simulink model "foc_current_estimator_test"  (R2021b)
settings: Solver=FixedStepDiscrete  StartTime=0.0  StopTime=6  FixedStep=Tsw  RelTol=1e-3
undefined symbols (not defined in the file): B, current_ki, current_kp, DiscIntNeverNeededParam, Ibase, id_ref, iq_ref, J, k1_sta, k2_sta, Ks, load_torque, Ls, qpll, Rs, sigmoid_a, speed_ki, speed_kp, Ts_speed, Tsw, Vbase, Vdc, w_base
libraries: mcbcontrolslib x6, simulink_extras x2, mcbplantlib x1, autolibpmsmexterior x1
settings Model: Creator=gary  LastModifiedBy=goldf
settings DebuggingCC: SFMachineParentedDataDiag=warning

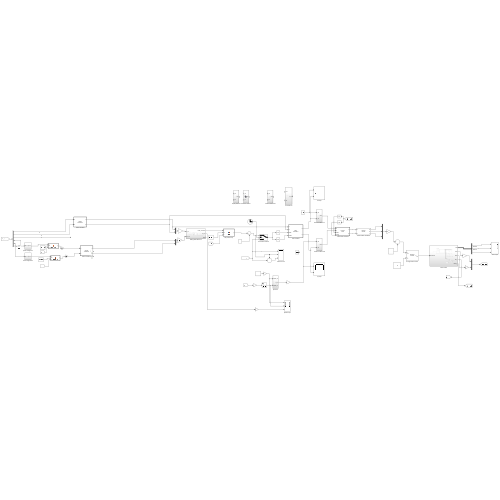
[thumbnail: Simulink's stored preview of the top-level diagram]
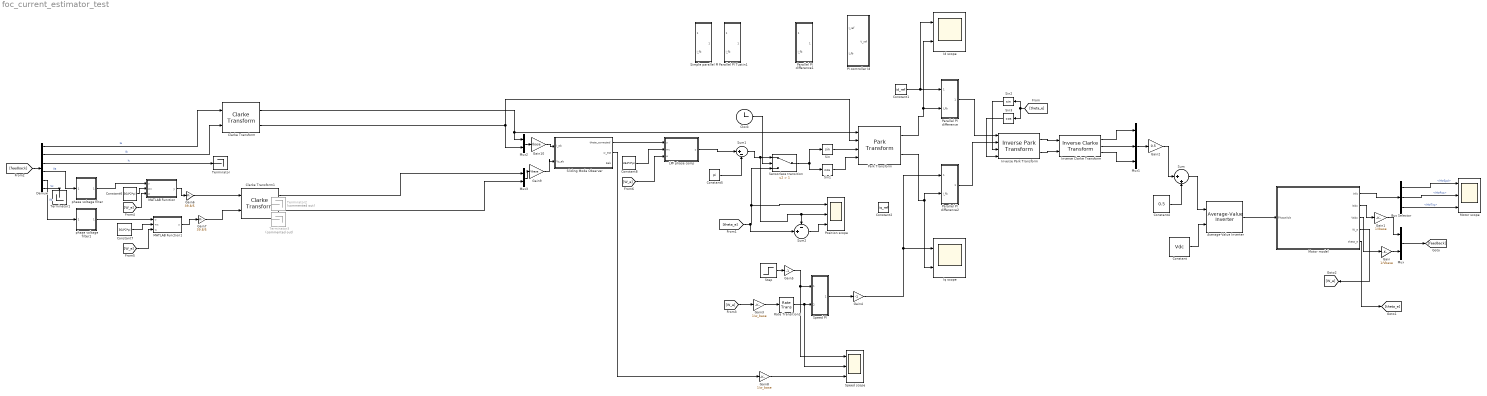
== system foc_current_estimator_test ==
  Average-Value Inverter : mcbplantlib/Average-Value Inverter
  Bus Selector : BusSelector  OutputSignals=MtrSpd,MtrPos,MtrTrq
  Clarke Transform : mcbcontrolslib/Clarke Transform  VariantControl=Variant2
  Clarke Transform1 : mcbcontrolslib/Clarke Transform  VariantControl=Variant2
  Clock : Clock
  Constant : Constant  Value=Vdc
  Constant1 : Constant  Value=id_ref
  Constant2 : Constant  Value=iq_ref
  Constant4 : Constant  Value=0.5
  Constant5 : Constant  Value=pi
  Constant6 : Constant  Value=364*2*pi
  Constant7 : Constant  Value=364*2*pi
  Constant8 : Constant  Value=364*2*pi
  Demux : Demux  Outputs=6
  Gain : Gain  Gain=1/Vbase
  Gain1 : Gain  Gain=1/Ibase
  Gain10 : Gain  Gain=Ibase
  Gain2 : Gain  Gain=0.5
  Gain3 : Gain  Gain=1/w_base
  Gain4 : Gain  Gain=-1
  Gain5 : Gain  Gain=-1
  Gain6 : Gain  Gain=39.8/5
  Gain7 : Gain  Gain=39.8/5
  Gain8 : Gain  Gain=1/w_base
  Gain9 : Gain  Gain=Vbase
  Id scope : Scope  NumInputPorts=2
  Inverse Clarke Transform : mcbcontrolslib/Inverse Clarke Transform
      settings: SourceProductBaseCode=MT
  Inverse Park Transform : mcbcontrolslib/Inverse Park Transform  AxisAlignment=D-axis
  Iq scope : Scope  NumInputPorts=2
  LPF phase comp : MATLAB Function  TreatAsAtomicUnit=on
  MATLAB Function : MATLAB Function  TreatAsAtomicUnit=on
  MATLAB Function1 : MATLAB Function  TreatAsAtomicUnit=on
  Motor model : Subsystem
  Motor scope : Scope  NumInputPorts=3
  Mux : Mux  Inputs=2
  Mux1 : Mux  Inputs=3
  Mux2 : Mux  Inputs=2
  Mux3 : Mux  Inputs=2
  PI controller Id : Subsystem
  Parallel PI Tustin1 : Subsystem
  Parallel PI difference : Subsystem
  Parallel PI difference1 : Subsystem
  Parallel PI difference2 : Subsystem
  Park Transform : mcbcontrolslib/Park Transform  AxisAlignment=D-axis
      settings: SourceProductBaseCode=MT
  Position scope : Scope  NumInputPorts=3
  Rate Transition2 : RateTransition  OutPortSampleTime=Ts_speed
  Sensorless transition : Switch  Criteria=u2 > Threshold  Threshold=1
  Simple parallel PI : Subsystem
  Sin : Trigonometry
  Sin1 : Trigonometry  Operator=cos
  Sin2 : Trigonometry
  Sin3 : Trigonometry  Operator=cos
  Sliding Mode Observer : Subsystem
  Speed PI : Subsystem
  Speed scope : Scope  NumInputPorts=3
  Step : Step  Time=3  Before=0.4  After=0.4  SampleTime=0
  Sum : Sum  Inputs=|++
  Sum1 : Sum  Inputs=|+-
  Sum2 : Sum  Inputs=-+|
  Terminator : Terminator
  Terminator1 : Terminator
  Terminator2 : Terminator  Commented=on
  Terminator3 : Terminator  Commented=on
  phase voltage filter : Subsystem
  phase voltage filter1 : Subsystem
  wires:
  Constant/1 -> Average-Value Inverter/2
  Motor model/1(Info) -> Bus Selector/1
  Bus Selector/2 -> Motor scope/2  "<MtrPos>"
  Bus Selector/3 -> Motor scope/3  "<MtrTrq>"
  Mux/1 -> [feedback]
  [feedback] -> Demux/1
  Demux/3 -> Terminator/1  "Ic"
  Demux/1 -> Clarke Transform/1  "Ia"
  Demux/2 -> Clarke Transform/2  "Ib"
  Park Transform/1 -> Parallel PI difference/2(I_fb), Id scope/2
  Park Transform/2 -> Parallel PI difference2/2(I_fb), Iq scope/2
  Constant1/1 -> Parallel PI difference/1(I_ref), Id scope/1
  Parallel PI difference/1(Vref) -> Inverse Park Transform/1
  Parallel PI difference2/1(Vref) -> Inverse Park Transform/2
  [theta_e] -> Sin2/1, Sin3/1
  Sin2/1 -> Inverse Park Transform/3
  Sin3/1 -> Inverse Park Transform/4
  Inverse Park Transform/1 -> Inverse Clarke Transform/1
  Inverse Park Transform/2 -> Inverse Clarke Transform/2
  Inverse Clarke Transform/2 -> Mux1/2
  Inverse Clarke Transform/3 -> Mux1/3
  Inverse Clarke Transform/1 -> Mux1/1
  Average-Value Inverter/1 -> Motor model/1(PhaseVolt)
  Motor model/2(Iabc) -> Gain1/1
  Gain1/1 -> Mux/1
  Motor model/3(Vabc) -> Gain/1
  Demux/6 -> Terminator1/1  "Vc"
  Clarke Transform/1 -> Mux2/1, Park Transform/1
  Clarke Transform/2 -> Mux2/2, Park Transform/2
  Sin/1 -> Park Transform/3
  Sin1/1 -> Park Transform/4
  Motor model/5(theta_e) -> [theta_e]
  Gain/1 -> Mux/2
  Mux1/1 -> Gain2/1
  Gain2/1 -> Sum/1
  Sum/1 -> Average-Value Inverter/1
  Constant4/1 -> Sum/2
  [theta_e] -> Sum2/2, Position scope/1, Sensorless transition/3
  Bus Selector/1 -> Motor scope/1  "<MtrSpd>"
  Clock/1 -> Sensorless transition/2
  Sensorless transition/1 -> Sin1/1, Sin/1
  Sum1/1 -> Sum2/1, Position scope/2, Sensorless transition/1
  Constant5/1 -> Sum1/2
  [W_e] -> Gain3/1
  Gain5/1 -> Speed scope/1, Speed PI/1(Speed_ref)
  Rate Transition2/1 -> Speed scope/2, Speed PI/2(Speed_fb)
  Step/1 -> Gain5/1
  Speed PI/1(I_ref) -> Gain4/1
  Gain3/1 -> Rate Transition2/1
  Motor model/4(W_e) -> [W_e]
  Gain4/1 -> Parallel PI difference2/1(I_ref), Iq scope/1
  [W_e] -> MATLAB Function/3(w)
  Constant6/1 -> MATLAB Function/2(wc)
  MATLAB Function/1(y) -> Gain6/1
  phase voltage filter/1(lpf out) -> MATLAB Function/1(u)
  phase voltage filter1/1(lpf out) -> MATLAB Function1/1(u)
  Constant7/1 -> MATLAB Function1/2(wc)
  [W_e] -> MATLAB Function1/3(w)
  MATLAB Function1/1(y) -> Gain7/1
  Demux/4 -> phase voltage filter/1(lpf in)  "Va"
  Demux/5 -> phase voltage filter1/1(lpf in)  "Vb"
  Constant8/1 -> LPF phase comp/2(wc)
  [W_e] -> LPF phase comp/3(w)
  Sliding Mode Observer/2(w_est) -> Gain8/1
  Gain8/1 -> Speed scope/3
  Mux2/1 -> Gain10/1
  Gain10/1 -> Sliding Mode Observer/1(I_ab)
  Mux3/1 -> Gain9/1
  Gain9/1 -> Sliding Mode Observer/2(Vs_ab)
  Sum2/1 -> Position scope/3
  Clarke Transform1/1 -> Mux3/1
  Clarke Transform1/2 -> Mux3/2
  Gain6/1 -> Clarke Transform1/1
  Gain7/1 -> Clarke Transform1/2
  Sliding Mode Observer/1(theta_corrected) -> LPF phase comp/1(u)
  LPF phase comp/1(y) -> Sum1/1

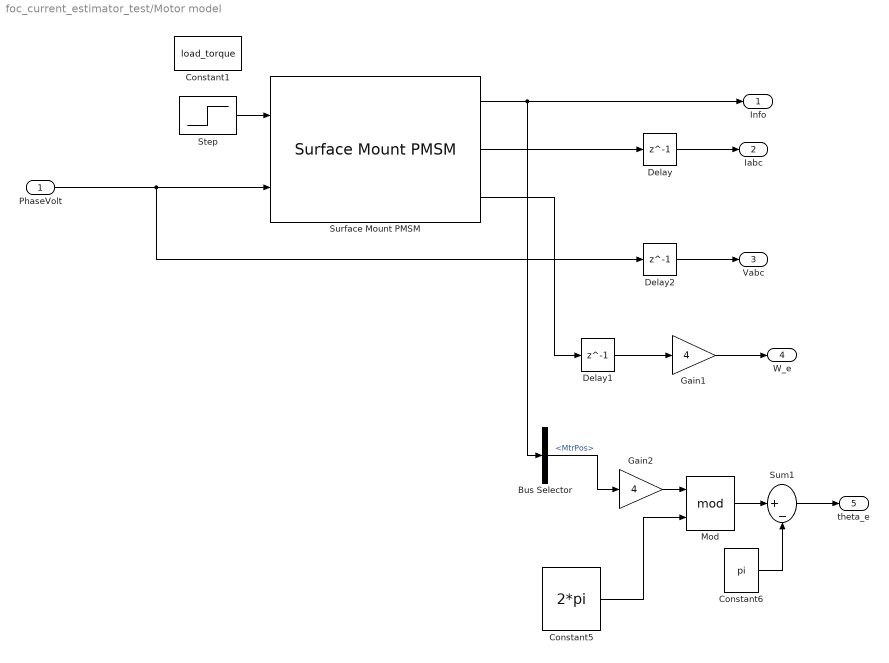
== system foc_current_estimator_test/Motor model ==
  PhaseVolt : Inport
  Bus Selector : BusSelector  OutputSignals=MtrPos
  Constant1 : Constant  Value=load_torque
  Constant5 : Constant  Value=2*pi
  Constant6 : Constant  Value=pi
  Delay : Delay  DelayLength=1  InitialCondition=0
  Delay1 : Delay  DelayLength=1  InitialCondition=0
  Delay2 : Delay  DelayLength=1  InitialCondition=0
  Gain1 : Gain  Gain=4
  Gain2 : Gain  Gain=4
  Mod : Math  Operator=mod  SaturateOnIntegerOverflow=on
  Step : Step  Time=3  Before=-0.02  After=-0.4  SampleTime=0
  Sum1 : Sum  Inputs=|+-
  Surface Mount PMSM : autolibpmsmexterior/Surface Mount PMSM  port_config=Torque  sim_type=Discrete  Ts=Tsw  P=4  Rs=1.5*Rs  Ldq_=0.3*Ls  KConstText=Permanent flux linkage constant (lambda_pm):  lambda_pm=lambda  Ke=159.9771  Kt=1.323  mechanical=[J, B, 0]  idq0=[0 0]  theta_init=0  omega_init=-100  KConst=lambda  lambda_pm_calc=lambda  RefBlkName='autolibpmsmexterior/Surface Mount PMSM'  aMode=5  Ldq="[0.0017      0.0017]"
      settings: SourceProductBaseCode=PW,DR,MT,UV,VE
  Info : Outport
  Iabc : Outport  Port=2
  Vabc : Outport  Port=3
  W_e : Outport  Port=4
  theta_e : Outport  Port=5
  wires:
  Surface Mount PMSM/1 -> Info/1, Bus Selector/1
  Surface Mount PMSM/2 -> Delay/1
  PhaseVolt/1 -> Delay2/1, Surface Mount PMSM/2
  Step/1 -> Surface Mount PMSM/1
  Surface Mount PMSM/3 -> Delay1/1
  Delay/1 -> Iabc/1
  Bus Selector/1 -> Gain2/1  "<MtrPos>"
  Gain2/1 -> Mod/1
  Constant5/1 -> Mod/2
  Sum1/1 -> theta_e/1
  Mod/1 -> Sum1/1
  Constant6/1 -> Sum1/2
  Delay1/1 -> Gain1/1
  Gain1/1 -> W_e/1
  Delay2/1 -> Vabc/1

== system foc_current_estimator_test/PI controller Id ==
  I_ref : Inport
  I_fb : Inport  Port=2
  Constant1 : Constant  Value=0
  Constant2 : Constant  Value=current_kp
  Constant3 : Constant  Value=current_ki*Tsw
  Constant4 : Constant  Value=0
  Discrete PI Controller with anti-windup & reset : mcbcontrolslib/Discrete PI Controller  with anti-windup & reset  UpperSaturationLimit=1  LowerSaturationLimit=-1
      settings: SourceProductBaseCode=MT
  Sum : Sum  Inputs=|+-
  V_ref : Outport
  wires:
  I_ref/1 -> Sum/1
  Constant4/1 -> Discrete PI Controller with anti-windup & reset/5
  Discrete PI Controller with anti-windup & reset/1 -> V_ref/1
  Constant1/1 -> Discrete PI Controller with anti-windup & reset/4
  I_fb/1 -> Sum/2
  Constant2/1 -> Discrete PI Controller with anti-windup & reset/2
  Sum/1 -> Discrete PI Controller with anti-windup & reset/1
  Constant3/1 -> Discrete PI Controller with anti-windup & reset/3

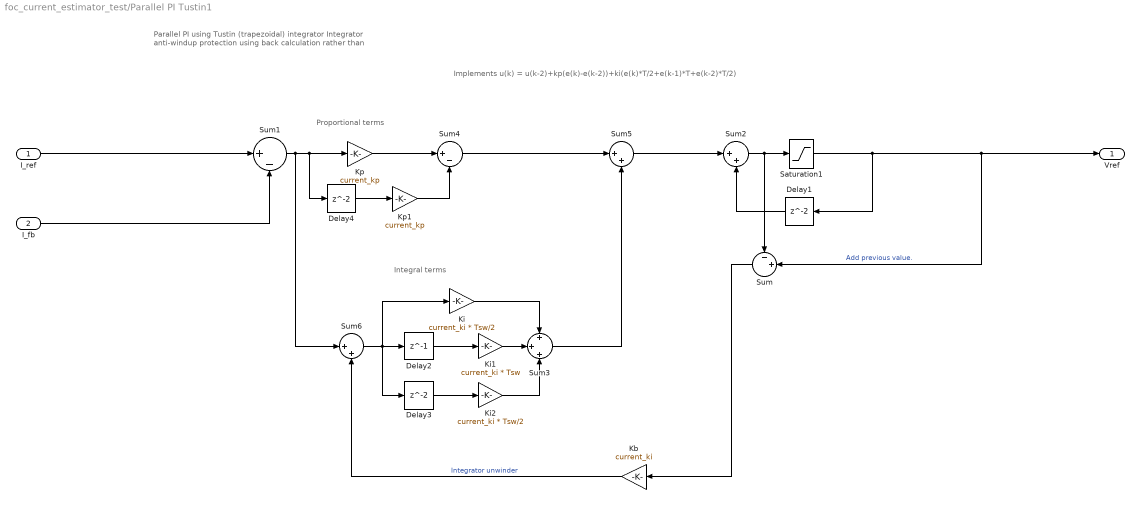
== system foc_current_estimator_test/Parallel PI Tustin1 ==
  note: Implements u(k) = u(k-2)+kp(e(k)-e(k-2))+ki(e(k)*T/2+e(k-1)*T+e(k-2)*T/2)
  note: Integral terms
  note: Proportional terms
  note: Parallel PI using Tustin (trapezoidal) integrator
      | Integrator anti-windup protection using back calculation
      | rather than
  I_ref : Inport
  I_fb : Inport  Port=2
  Delay1 : Delay  InitialCondition=0
  Delay2 : Delay  DelayLength=1  InitialCondition=0
  Delay3 : Delay  InitialCondition=0
  Delay4 : Delay  InitialCondition=0
  Kb : Gain  Gain=current_ki
  Ki : Gain  Gain=current_ki * Tsw/2
  Ki1 : Gain  Gain=current_ki * Tsw
  Ki2 : Gain  Gain=current_ki * Tsw/2
  Kp : Gain  Gain=current_kp
  Kp1 : Gain  Gain=current_kp
  Saturation1 : Saturate  UpperLimit=1  LowerLimit=-1
  Sum : Sum  Inputs=-+|
  Sum1 : Sum  Inputs=|+-
  Sum2 : Sum  Inputs=|++
  Sum3 : Sum  Inputs=+|+|+
  Sum4 : Sum  Inputs=|+-
  Sum5 : Sum  Inputs=|++
  Sum6 : Sum  Inputs=|++
  Vref : Outport
  wires:
  Sum1/1 -> Sum6/1, Delay4/1, Kp/1
  I_fb/1 -> Sum1/2
  I_ref/1 -> Sum1/1
  Kp/1 -> Sum4/1
  Delay1/1 -> Sum2/2
  Sum2/1 -> Sum/1, Saturation1/1
  Sum/1 -> Kb/1
  Delay2/1 -> Ki1/1
  Delay3/1 -> Ki2/1
  Delay4/1 -> Kp1/1
  Kp1/1 -> Sum4/2
  Ki1/1 -> Sum3/2
  Ki/1 -> Sum3/1
  Ki2/1 -> Sum3/3
  Sum4/1 -> Sum5/1
  Sum6/1 -> Delay3/1, Delay2/1, Ki/1
  Sum3/1 -> Sum5/2
  Sum5/1 -> Sum2/1
  Kb/1 -> Sum6/2  "Integrator unwinder"
  Saturation1/1 -> Sum/2, Vref/1, Delay1/1  "Add previous value."

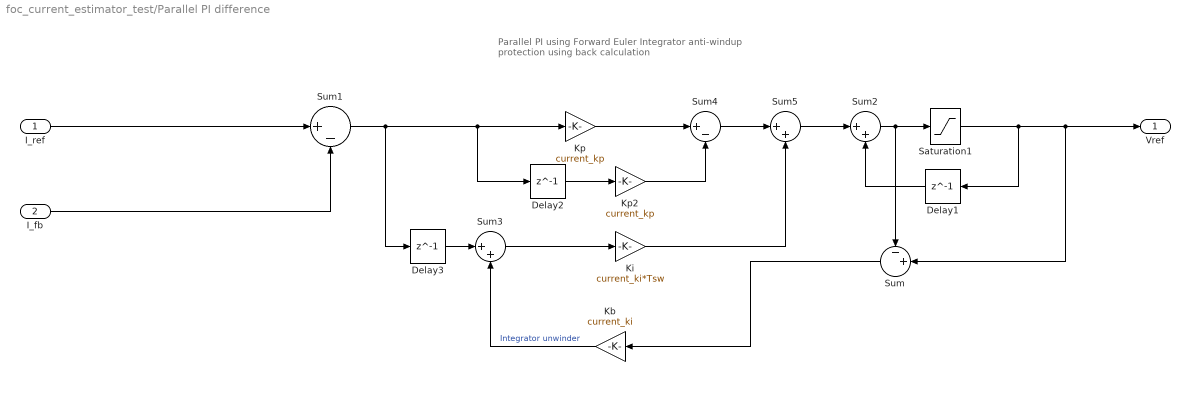
== system foc_current_estimator_test/Parallel PI difference ==
  note: Parallel PI using Forward Euler
      | Integrator anti-windup protection using back calculation
  I_ref : Inport
  I_fb : Inport  Port=2
  Delay1 : Delay  DelayLength=1  InitialCondition=0
  Delay2 : Delay  DelayLength=1  InitialCondition=0
  Delay3 : Delay  DelayLength=1  InitialCondition=0
  Kb : Gain  Gain=current_ki
  Ki : Gain  Gain=current_ki*Tsw
  Kp : Gain  Gain=current_kp
  Kp2 : Gain  Gain=current_kp
  Saturation1 : Saturate  UpperLimit=1  LowerLimit=0
  Sum : Sum  Inputs=-+|
  Sum1 : Sum  Inputs=|+-
  Sum2 : Sum  Inputs=|++
  Sum3 : Sum  Inputs=|++
  Sum4 : Sum  Inputs=|+-
  Sum5 : Sum  Inputs=|++
  Vref : Outport
  wires:
  I_fb/1 -> Sum1/2
  I_ref/1 -> Sum1/1
  Sum1/1 -> Delay2/1, Kp/1, Delay3/1
  Kp/1 -> Sum4/1
  Delay1/1 -> Sum2/2
  Sum2/1 -> Saturation1/1, Sum/1
  Saturation1/1 -> Sum/2, Vref/1, Delay1/1
  Kb/1 -> Sum3/2  "Integrator unwinder"
  Sum/1 -> Kb/1
  Delay2/1 -> Kp2/1
  Kp2/1 -> Sum4/2
  Sum3/1 -> Ki/1
  Delay3/1 -> Sum3/1
  Sum4/1 -> Sum5/1
  Ki/1 -> Sum5/2
  Sum5/1 -> Sum2/1

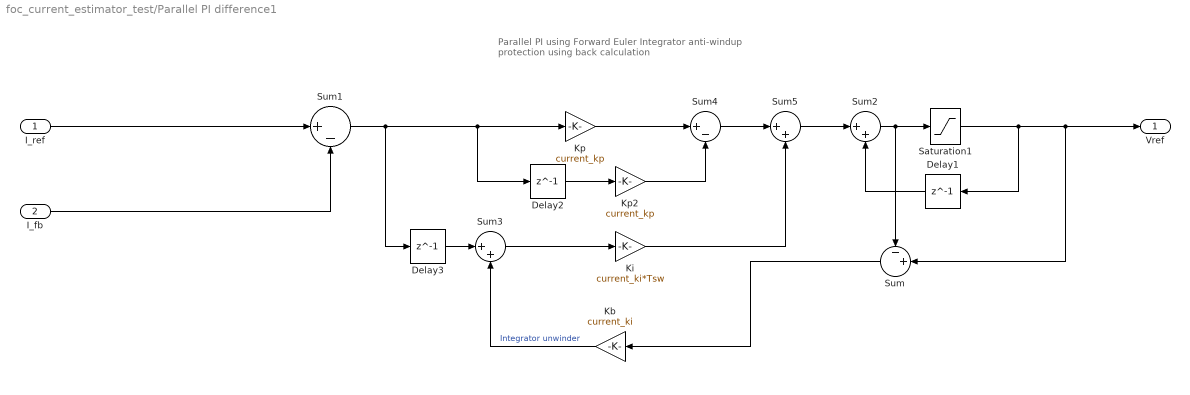
== system foc_current_estimator_test/Parallel PI difference1 ==
  note: Parallel PI using Forward Euler
      | Integrator anti-windup protection using back calculation
  I_ref : Inport
  I_fb : Inport  Port=2
  Delay1 : Delay  DelayLength=1  InitialCondition=0
  Delay2 : Delay  DelayLength=1  InitialCondition=0
  Delay3 : Delay  DelayLength=1  InitialCondition=0
  Kb : Gain  Gain=current_ki
  Ki : Gain  Gain=current_ki*Tsw
  Kp : Gain  Gain=current_kp
  Kp2 : Gain  Gain=current_kp
  Saturation1 : Saturate  UpperLimit=1  LowerLimit=0
  Sum : Sum  Inputs=-+|
  Sum1 : Sum  Inputs=|+-
  Sum2 : Sum  Inputs=|++
  Sum3 : Sum  Inputs=|++
  Sum4 : Sum  Inputs=|+-
  Sum5 : Sum  Inputs=|++
  Vref : Outport
  wires:
  I_fb/1 -> Sum1/2
  I_ref/1 -> Sum1/1
  Sum1/1 -> Delay2/1, Kp/1, Delay3/1
  Kp/1 -> Sum4/1
  Delay1/1 -> Sum2/2
  Sum2/1 -> Saturation1/1, Sum/1
  Saturation1/1 -> Sum/2, Vref/1, Delay1/1
  Kb/1 -> Sum3/2  "Integrator unwinder"
  Sum/1 -> Kb/1
  Delay2/1 -> Kp2/1
  Kp2/1 -> Sum4/2
  Sum3/1 -> Ki/1
  Delay3/1 -> Sum3/1
  Sum4/1 -> Sum5/1
  Ki/1 -> Sum5/2
  Sum5/1 -> Sum2/1

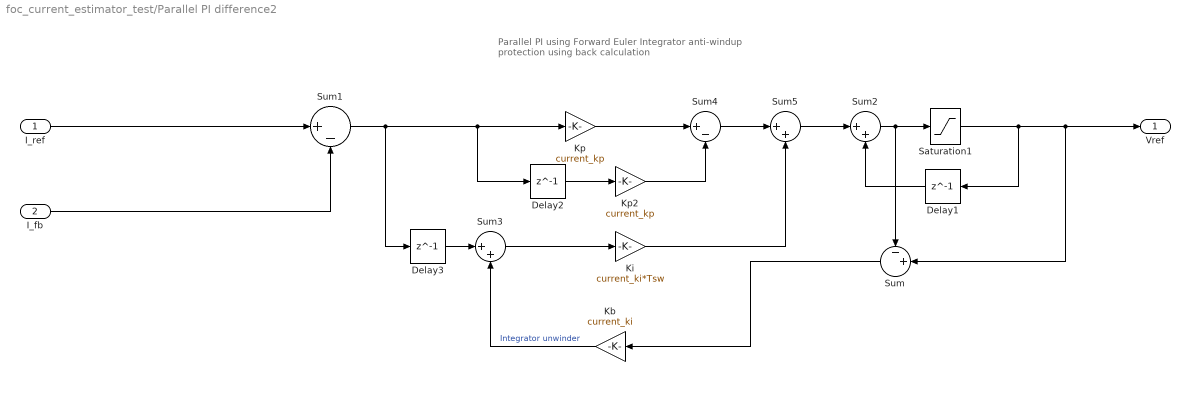
== system foc_current_estimator_test/Parallel PI difference2 ==
  note: Parallel PI using Forward Euler
      | Integrator anti-windup protection using back calculation
  I_ref : Inport
  I_fb : Inport  Port=2
  Delay1 : Delay  DelayLength=1  InitialCondition=0
  Delay2 : Delay  DelayLength=1  InitialCondition=0
  Delay3 : Delay  DelayLength=1  InitialCondition=0
  Kb : Gain  Gain=current_ki
  Ki : Gain  Gain=current_ki*Tsw
  Kp : Gain  Gain=current_kp
  Kp2 : Gain  Gain=current_kp
  Saturation1 : Saturate  UpperLimit=1  LowerLimit=0
  Sum : Sum  Inputs=-+|
  Sum1 : Sum  Inputs=|+-
  Sum2 : Sum  Inputs=|++
  Sum3 : Sum  Inputs=|++
  Sum4 : Sum  Inputs=|+-
  Sum5 : Sum  Inputs=|++
  Vref : Outport
  wires:
  I_fb/1 -> Sum1/2
  I_ref/1 -> Sum1/1
  Sum1/1 -> Delay2/1, Kp/1, Delay3/1
  Kp/1 -> Sum4/1
  Delay1/1 -> Sum2/2
  Sum2/1 -> Saturation1/1, Sum/1
  Saturation1/1 -> Sum/2, Vref/1, Delay1/1
  Kb/1 -> Sum3/2  "Integrator unwinder"
  Sum/1 -> Kb/1
  Delay2/1 -> Kp2/1
  Kp2/1 -> Sum4/2
  Sum3/1 -> Ki/1
  Delay3/1 -> Sum3/1
  Sum4/1 -> Sum5/1
  Ki/1 -> Sum5/2
  Sum5/1 -> Sum2/1

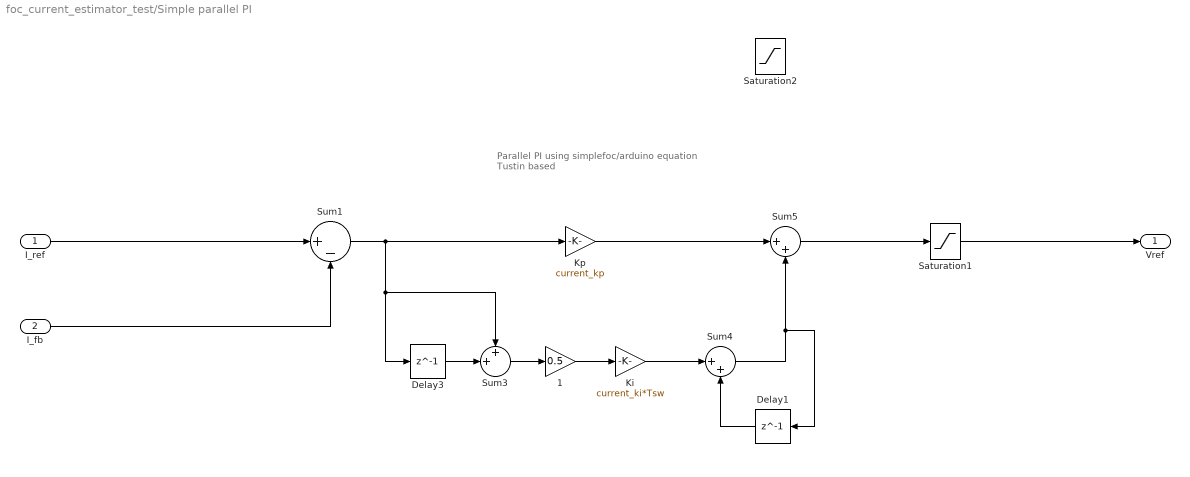
== system foc_current_estimator_test/Simple parallel PI ==
  note: Parallel PI using simplefoc/arduino equation
      | Tustin based
  I_ref : Inport
  I_fb : Inport  Port=2
  1 : Gain  Gain=0.5
  Delay1 : Delay  DelayLength=1  InitialCondition=0
  Delay3 : Delay  DelayLength=1  InitialCondition=0
  Ki : Gain  Gain=current_ki*Tsw
  Kp : Gain  Gain=current_kp
  Saturation1 : Saturate  UpperLimit=1  LowerLimit=0
  Saturation2 : Saturate  UpperLimit=1  LowerLimit=0
  Sum1 : Sum  Inputs=|+-
  Sum3 : Sum  Inputs=++|
  Sum4 : Sum  Inputs=|++
  Sum5 : Sum  Inputs=|++
  Vref : Outport
  wires:
  I_fb/1 -> Sum1/2
  I_ref/1 -> Sum1/1
  Sum5/1 -> Saturation1/1
  Saturation1/1 -> Vref/1
  Sum3/1 -> 1/1
  Kp/1 -> Sum5/1
  Delay3/1 -> Sum3/2
  Sum1/1 -> Kp/1, Sum3/1, Delay3/1
  1/1 -> Ki/1
  Ki/1 -> Sum4/1
  Sum4/1 -> Delay1/1, Sum5/2
  Delay1/1 -> Sum4/2

== system foc_current_estimator_test/Sliding Mode Observer ==
  I_ab : Inport
  Vs_ab : Inport  Port=2
  Constant10 : Constant  Value=qpll.kp
  Constant9 : Constant  Value=qpll.ki
  Demux1 : Demux  Outputs=2
  QPLL : Subsystem
  Reversal 180 phase shift : Subsystem
  SMO bemf estimator1 : Subsystem
  SMO bemf estimator3 : Subsystem  Commented=on
  theta_corrected : Outport
  w_est : Outport  Port=2
  Eab : Outport  Port=3
  wires:
  SMO bemf estimator1/1(E_ab) -> Eab/1, Demux1/1
  Reversal 180 phase shift/1(theta_corrected) -> theta_corrected/1
  Constant9/1 -> QPLL/2(ki)
  Vs_ab/1 -> SMO bemf estimator1/2(Vs_ab)
  QPLL/1(theta_est) -> Reversal 180 phase shift/1(theta_uncorrected)
  Constant10/1 -> QPLL/1(kp)
  QPLL/2(w) -> w_est/1, Reversal 180 phase shift/2(W_est)
  Demux1/2 -> QPLL/4(E_beta)
  Demux1/1 -> QPLL/3(E_alpha)
  I_ab/1 -> SMO bemf estimator1/1(I_ab)

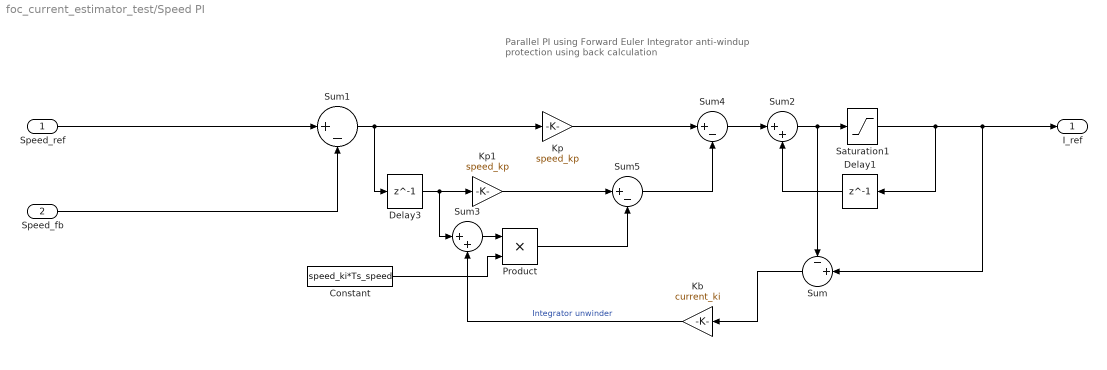
== system foc_current_estimator_test/Speed PI ==
  note: Parallel PI using Forward Euler
      | Integrator anti-windup protection using back calculation
  Speed_ref : Inport
  Speed_fb : Inport  Port=2
  Constant : Constant  Value=speed_ki*Ts_speed
  Delay1 : Delay  DelayLength=1  InitialCondition=0
  Delay3 : Delay  DelayLength=1  InitialCondition=0
  Kb : Gain  Gain=current_ki
  Kp : Gain  Gain=speed_kp
  Kp1 : Gain  Gain=speed_kp
  Product : Product
  Saturation1 : Saturate  UpperLimit=1  LowerLimit=-1
  Sum : Sum  Inputs=-+|
  Sum1 : Sum  Inputs=|+-
  Sum2 : Sum  Inputs=|++
  Sum3 : Sum  Inputs=|++
  Sum4 : Sum  Inputs=|+-
  Sum5 : Sum  Inputs=|+-
  I_ref : Outport
  wires:
  Sum1/1 -> Delay3/1, Kp/1
  Speed_fb/1 -> Sum1/2
  Speed_ref/1 -> Sum1/1
  Constant/1 -> Product/2
  Delay3/1 -> Kp1/1, Sum3/1
  Kp1/1 -> Sum5/1
  Kp/1 -> Sum4/1
  Delay1/1 -> Sum2/2
  Sum4/1 -> Sum2/1
  Sum2/1 -> Sum/1, Saturation1/1
  Sum5/1 -> Sum4/2
  Product/1 -> Sum5/2
  Sum3/1 -> Product/1
  Kb/1 -> Sum3/2  "Integrator unwinder"
  Sum/1 -> Kb/1
  Saturation1/1 -> Sum/2, I_ref/1, Delay1/1

== system foc_current_estimator_test/phase voltage filter ==
  lpf in : Inport
  Instaspin lpf tf : simulink_extras/Additional Discrete/Discrete Transfer Fcn (with initial outputs)  N=[0.006918, 0.006659]  D=[1 -0.8919]  U0=[1]  Y0=0  TS=-1
      settings: SourceProductBaseCode=SL
  Rate Transition1 : RateTransition  OutPortSampleTime=Tsw
  lpf out : Outport
  wires:
  Rate Transition1/1 -> Instaspin lpf tf/1
  Instaspin lpf tf/1 -> lpf out/1
  lpf in/1 -> Rate Transition1/1

== system foc_current_estimator_test/phase voltage filter1 ==
  lpf in : Inport
  Instaspin lpf tf : simulink_extras/Additional Discrete/Discrete Transfer Fcn (with initial outputs)  N=[0.006918, 0.006659]  D=[1 -0.8919]  U0=[1]  Y0=0  TS=-1
      settings: SourceProductBaseCode=SL
  Rate Transition1 : RateTransition  OutPortSampleTime=Tsw
  lpf out : Outport
  wires:
  Rate Transition1/1 -> Instaspin lpf tf/1
  Instaspin lpf tf/1 -> lpf out/1
  lpf in/1 -> Rate Transition1/1

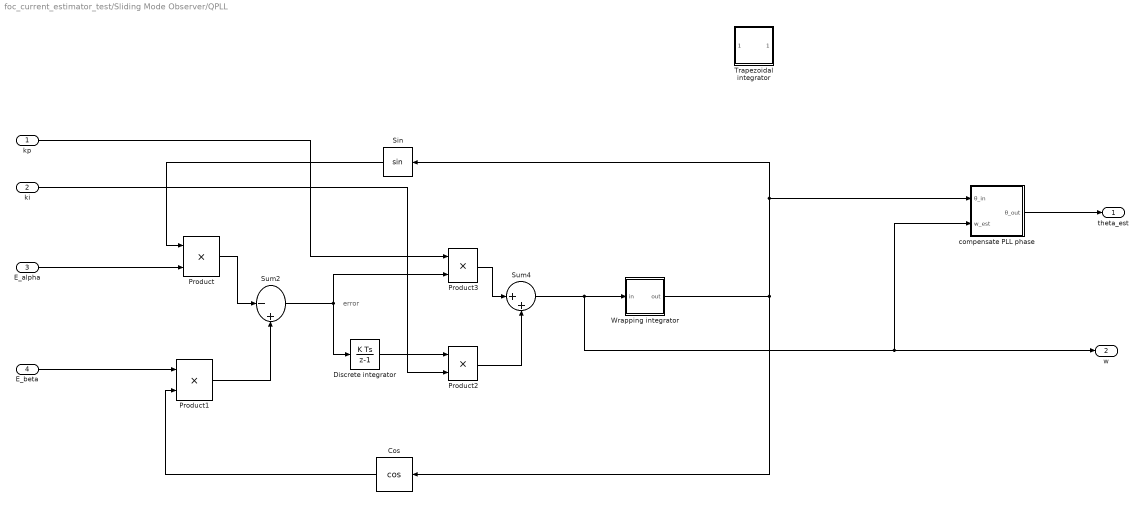
== system foc_current_estimator_test/Sliding Mode Observer/QPLL ==
  note: error
  kp : Inport
  ki : Inport  Port=2
  E_alpha : Inport  Port=3
  E_beta : Inport  Port=4
  Cos : Trigonometry  Operator=cos
  Discrete integrator : DiscreteIntegrator  SampleTime=-1  ICPrevOutput=DiscIntNeverNeededParam  ICPrevScaledInput=DiscIntNeverNeededParam
  Product{,1..3} (4 alike) : Product
  Sin : Trigonometry
  Sum2 : Sum  Inputs=|-+
  Sum4 : Sum  Inputs=|++
  Trapezoidal integrator : Subsystem
  Wrapping integrator : Subsystem
      mask help: The integrator uses the Forward Euler method and wraps its state between 0 and 2*pi.
  compensate PLL phase : Subsystem
  theta_est : Outport
  w : Outport  Port=2
  wires:
  Sin/1 -> Product/1
  Cos/1 -> Product1/2
  Sum4/1 -> Wrapping integrator/1(in), compensate PLL phase/2(w_est), w/1
  Product1/1 -> Sum2/2
  Product/1 -> Sum2/1
  kp/1 -> Product3/1
  Discrete integrator/1 -> Product2/1
  ki/1 -> Product2/2
  Product3/1 -> Sum4/1
  Product2/1 -> Sum4/2
  compensate PLL phase/1(θ_out) -> theta_est/1
  E_alpha/1 -> Product/2
  E_beta/1 -> Product1/1
  Wrapping integrator/1(out) -> Cos/1, Sin/1, compensate PLL phase/1(θ_in)
  Sum2/1 -> Discrete integrator/1, Product3/2

== system foc_current_estimator_test/Sliding Mode Observer/Reversal 180 phase shift ==
  theta_uncorrected : Inport
  W_est : Inport  Port=2
  Constant2 : Constant  Value=0
  Constant3 : Constant  Value=pi
  Constant4 : Constant  Value=2*pi
  Mod : Math  Operator=mod  SaturateOnIntegerOverflow=on
  Sign : Signum
  Sum : Sum  Inputs=|++
  Switch : Switch  Criteria=u2 > Threshold
  theta_corrected : Outport
  wires:
  Constant2/1 -> Switch/1
  Constant3/1 -> Switch/3
  Sum/1 -> Mod/1
  Constant4/1 -> Mod/2
  Switch/1 -> Sum/1
  Sign/1 -> Switch/2
  Mod/1 -> theta_corrected/1
  theta_uncorrected/1 -> Sum/2
  W_est/1 -> Sign/1

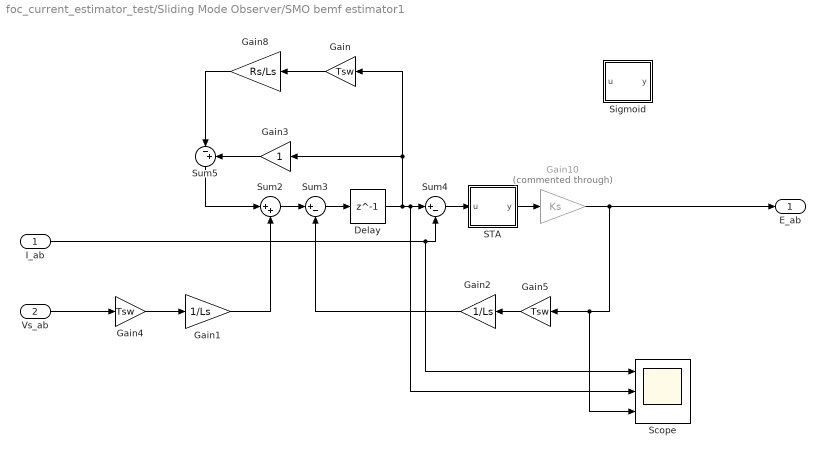
== system foc_current_estimator_test/Sliding Mode Observer/SMO bemf estimator1 ==
  I_ab : Inport
  Vs_ab : Inport  Port=2
  Delay : Delay  DelayLength=1  InitialCondition=0
  Gain : Gain  Gain=Tsw
  Gain1 : Gain  Gain=1/Ls
  Gain10 : Gain  Commented=through  Gain=Ks
  Gain2 : Gain  Gain=1/Ls
  Gain3 : Gain
  Gain4 : Gain  Gain=Tsw
  Gain5 : Gain  Gain=Tsw
  Gain8 : Gain  Gain=Rs/Ls
  STA : Subsystem
      mask Display: plot(linspace(-1,1,100),(2./(1+exp(-10*linspace(-1,1,100))))-1)
  Scope : Scope  NumInputPorts=3
  Sigmoid : Subsystem
      mask Display: plot(linspace(-1,1,100),(2./(1+exp(-10*linspace(-1,1,100))))-1)
  Sum2 : Sum  Inputs=|++
  Sum3 : Sum  Inputs=|+-
  Sum4 : Sum  Inputs=|+-
  Sum5 : Sum  Inputs=|-+
  E_ab : Outport
  wires:
  Sum5/1 -> Sum2/1
  Gain8/1 -> Sum5/1
  Sum4/1 -> STA/1(u)
  Sum2/1 -> Sum3/1
  STA/1(y) -> Gain10/1
  Gain10/1 -> Scope/3, Gain5/1, E_ab/1
  Sum3/1 -> Delay/1
  Vs_ab/1 -> Gain4/1
  I_ab/1 -> Scope/1, Sum4/2
  Gain2/1 -> Sum3/2
  Gain/1 -> Gain8/1
  Gain5/1 -> Gain2/1
  Gain1/1 -> Sum2/2
  Gain4/1 -> Gain1/1
  Gain3/1 -> Sum5/2
  Delay/1 -> Gain3/1, Gain/1, Scope/2, Sum4/1

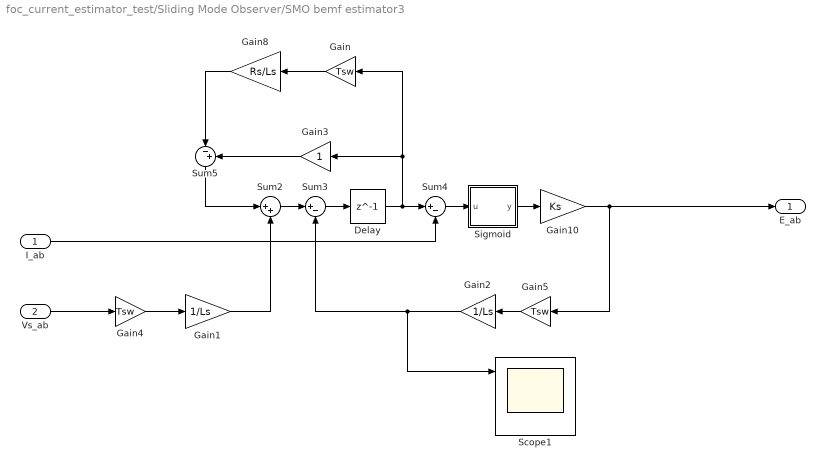
== system foc_current_estimator_test/Sliding Mode Observer/SMO bemf estimator3 ==
  I_ab : Inport
  Vs_ab : Inport  Port=2
  Delay : Delay  DelayLength=1  InitialCondition=0
  Gain : Gain  Gain=Tsw
  Gain1 : Gain  Gain=1/Ls
  Gain10 : Gain  Gain=Ks
  Gain2 : Gain  Gain=1/Ls
  Gain3 : Gain
  Gain4 : Gain  Gain=Tsw
  Gain5 : Gain  Gain=Tsw
  Gain8 : Gain  Gain=Rs/Ls
  Scope1 : Scope  NumInputPorts=3
  Sigmoid : Subsystem
      mask Display: plot(linspace(-1,1,100),(2./(1+exp(-10*linspace(-1,1,100))))-1)
  Sum2 : Sum  Inputs=|++
  Sum3 : Sum  Inputs=|+-
  Sum4 : Sum  Inputs=|+-
  Sum5 : Sum  Inputs=|-+
  E_ab : Outport
  wires:
  Sum5/1 -> Sum2/1
  Gain8/1 -> Sum5/1
  Sum4/1 -> Sigmoid/1(u)
  Sum2/1 -> Sum3/1
  Sigmoid/1(y) -> Gain10/1
  Gain10/1 -> Gain5/1, E_ab/1
  Sum3/1 -> Delay/1
  Vs_ab/1 -> Gain4/1
  Delay/1 -> Gain/1, Gain3/1, Sum4/1
  I_ab/1 -> Sum4/2
  Gain2/1 -> Scope1/1, Sum3/2
  Gain/1 -> Gain8/1
  Gain5/1 -> Gain2/1
  Gain1/1 -> Sum2/2
  Gain4/1 -> Gain1/1
  Gain3/1 -> Sum5/2

== system foc_current_estimator_test/Sliding Mode Observer/QPLL/Trapezoidal integrator ==
  Input : Inport
  Delay1 : Delay  DelayLength=1
  Delay2 : Delay  DelayLength=1
  Gain : Gain  Gain=Tsw
  Gain1 : Gain  Gain=0.5
  Math Function : Math  Operator=mod  SignedPower=on  OutputSignalType=real  SaturateOnIntegerOverflow=on
  Sum1 : Sum  Inputs=|++
  Sum3 : Sum  Inputs=|++
  cst : Constant  Value=2*pi  OutDataTypeStr=Inherit: Inherit via back propagation
  Output : Outport
  wires:
  cst/1 -> Math Function/2
  Sum3/1 -> Gain1/1
  Gain/1 -> Sum1/1
  Input/1 -> Delay2/1, Sum3/1
  Delay2/1 -> Sum3/2
  Gain1/1 -> Gain/1
  Math Function/1 -> Output/1, Delay1/1
  Sum1/1 -> Math Function/1
  Delay1/1 -> Sum1/2

== system foc_current_estimator_test/Sliding Mode Observer/QPLL/Wrapping integrator ==
  in : Inport
  Delay1 : Delay  DelayLength=1
  Gain : Gain  Gain=Tsw
  Math Function : Math  Operator=mod  SignedPower=on  OutputSignalType=real  SaturateOnIntegerOverflow=on
  Sum1 : Sum  Inputs=|++
  Weighted Sample Time : SampleTimeMath  TsampMathOp=*
  cst : Constant  Value=2*pi  OutDataTypeStr=Inherit: Inherit via back propagation
  out : Outport
  wires:
  in/1 -> Gain/1
  cst/1 -> Math Function/2
  Gain/1 -> Sum1/1
  Sum1/1 -> Math Function/1
  Delay1/1 -> Sum1/2
  Math Function/1 -> out/1, Delay1/1

== system foc_current_estimator_test/Sliding Mode Observer/QPLL/compensate PLL phase ==
  θ_in : Inport
  w_est : Inport  Port=2
  Constant : Constant  Value=2*pi
  Gain : Gain  Gain=pi/2
  Mod : Math  Operator=mod  SaturateOnIntegerOverflow=on
  Sign : Signum
  Sum : Sum  Inputs=|++
  θ_out : Outport
  wires:
  θ_in/1 -> Sum/1
  Sign/1 -> Gain/1
  w_est/1 -> Sign/1
  Gain/1 -> Sum/2
  Sum/1 -> Mod/1
  Constant/1 -> Mod/2
  Mod/1 -> θ_out/1

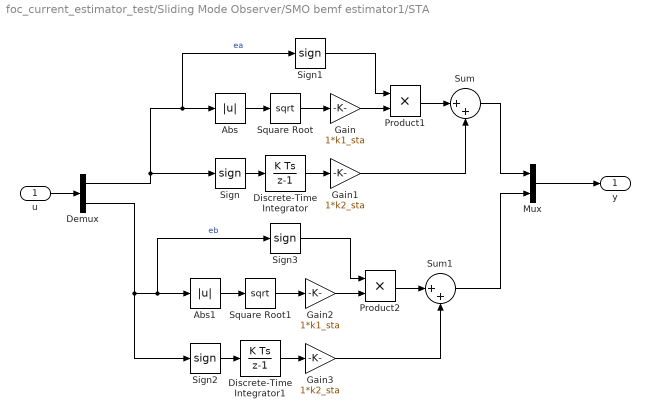
== system foc_current_estimator_test/Sliding Mode Observer/SMO bemf estimator1/STA ==
  u : Inport
  Abs : Abs
  Abs1 : Abs
  Demux : Demux  Outputs=2
  Discrete-Time Integrator : DiscreteIntegrator  SampleTime=-1  ICPrevOutput=DiscIntNeverNeededParam  ICPrevScaledInput=DiscIntNeverNeededParam
  Discrete-Time Integrator1 : DiscreteIntegrator  SampleTime=-1  ICPrevOutput=DiscIntNeverNeededParam  ICPrevScaledInput=DiscIntNeverNeededParam
  Gain : Gain  Gain=1*k1_sta
  Gain1 : Gain  Gain=1*k2_sta
  Gain2 : Gain  Gain=1*k1_sta
  Gain3 : Gain  Gain=1*k2_sta
  Mux : Mux  Inputs=2
  Product1 : Product
  Product2 : Product
  Sign{,1..3} (4 alike) : Signum
  Square Root : Sqrt  SaturateOnIntegerOverflow=on
  Square Root1 : Sqrt  SaturateOnIntegerOverflow=on
  Sum : Sum  Inputs=|++
  Sum1 : Sum  Inputs=|++
  y : Outport
  wires:
  Square Root/1 -> Gain/1
  Gain/1 -> Product1/2
  Sign1/1 -> Product1/1
  Abs/1 -> Square Root/1
  Product1/1 -> Sum/1
  Sign/1 -> Discrete-Time Integrator/1
  Discrete-Time Integrator/1 -> Gain1/1
  Gain1/1 -> Sum/2
  Sum/1 -> Mux/1
  u/1 -> Demux/1
  Demux/1 -> Sign1/1, Abs/1, Sign/1  "ea"
  Mux/1 -> y/1
  Abs1/1 -> Square Root1/1
  Sign3/1 -> Product2/1
  Demux/2 -> Sign2/1, Sign3/1, Abs1/1  "eb"
  Product2/1 -> Sum1/1
  Gain3/1 -> Sum1/2
  Square Root1/1 -> Gain2/1
  Gain2/1 -> Product2/2
  Sum1/1 -> Mux/2
  Sign2/1 -> Discrete-Time Integrator1/1
  Discrete-Time Integrator1/1 -> Gain3/1

== system foc_current_estimator_test/Sliding Mode Observer/SMO bemf estimator1/Sigmoid ==
  u : Inport
  Constant : Constant  Value=sigmoid_a
  Demux : Demux  Outputs=2
  Mux : Mux  Inputs=2
  sigmoid : MATLAB Function  TreatAsAtomicUnit=on
  sigmoid1 : MATLAB Function  TreatAsAtomicUnit=on
  y : Outport
  wires:
  Demux/2 -> sigmoid1/1(u)
  Demux/1 -> sigmoid/1(u)
  u/1 -> Demux/1
  sigmoid1/1(y) -> Mux/2
  sigmoid/1(y) -> Mux/1
  Mux/1 -> y/1
  Constant/1 -> sigmoid1/2(a), sigmoid/2(a)

== system foc_current_estimator_test/Sliding Mode Observer/SMO bemf estimator3/Sigmoid ==
  u : Inport
  Constant : Constant  Value=sigmoid_a
  Demux : Demux  Outputs=2
  Mux : Mux  Inputs=2
  sigmoid : MATLAB Function  TreatAsAtomicUnit=on
  sigmoid1 : MATLAB Function  TreatAsAtomicUnit=on
  y : Outport
  wires:
  Demux/2 -> sigmoid1/1(u)
  Demux/1 -> sigmoid/1(u)
  u/1 -> Demux/1
  sigmoid1/1(y) -> Mux/2
  sigmoid/1(y) -> Mux/1
  Mux/1 -> y/1
  Constant/1 -> sigmoid1/2(a), sigmoid/2(a)

== matlab function foc_current_estimator_test/MATLAB Function1 ==
  data: u input; y output; wc input; w input
function y = gain_comp(u, wc, w)
% Compensate for first order low-pass filter attentuation
% Using gain = 1 / (sqrt(1+(w/wc).^2));

y = u * sqrt(1+(w/wc).^2);

== matlab function foc_current_estimator_test/MATLAB Function ==
  data: u input; y output; wc input; w input
function y = gain_comp(u, wc, w)
% Compensate for first order low-pass filter attentuation
% Using gain = 1 / (sqrt(1+(w/wc).^2));

y = u * sqrt(1+(w/wc).^2);

== matlab function foc_current_estimator_test/LPF phase comp ==
  data: u input; y output; wc input; w input
function y = phase_comp(u, wc, w)
% Compensate for first order low-pass filter attentuation
% Using gain = 1 / (sqrt(1+(w/wc).^2));
% Note pole frequency is wc

lag = atan(w/wc);
y = u + lag;
y = mod(y,2*pi);

== matlab function foc_current_estimator_test/Sliding Mode Observer/SMO bemf estimator3/Sigmoid/sigmoid ==
  data: y output; u input; a input
function y = sigmoid(u,a)
% Sigmoid function instead of signum

y = (2/(1+exp(-a*u)))-1;

== matlab function foc_current_estimator_test/Sliding Mode Observer/SMO bemf estimator3/Sigmoid/sigmoid1 ==
  data: y output; u input; a input
function y = sigmoid(u,a)
% Sigmoid function instead of signum

y = (2/(1+exp(-a*u)))-1;

== matlab function foc_current_estimator_test/Sliding Mode Observer/SMO bemf estimator1/Sigmoid/sigmoid ==
  data: y output; u input; a input
function y = sigmoid(u,a)
% Sigmoid function instead of signum

y = (2/(1+exp(-a*u)))-1;

== matlab function foc_current_estimator_test/Sliding Mode Observer/SMO bemf estimator1/Sigmoid/sigmoid1 ==
  data: y output; u input; a input
function y = sigmoid(u,a)
% Sigmoid function instead of signum

y = (2/(1+exp(-a*u)))-1;
